simulink model "dev_AON_AOF_custom_detection_s_works"  (R2017b)
settings: Solver=ode5  StartTime=0.0  StopTime=20  FixedStep=0.025  RelTol=1e-3  EnableMultiTasking=on
undefined symbols (not defined in the file or in its folder): A1, B1
libraries: simulink x3
settings Model: Creator=b1048743  LastModifiedBy=Tom
settings DataIOCC: LimitDataPoints=on  SaveFormat=Array  SignalLoggingSaveFormat=ModelDataLogs  SignalLoggingName=sigsOut
settings OptimizationCC: BlockReduction=off  BooleanDataType=off
settings DebuggingCC: SaveWithParameterizedLinksMsg=none  UnderspecifiedInitializationDetection=Classic  MergeDetectMultiDrivingBlocksExec=none  SignalResolutionControl=TryResolveAllWithWarning  MultiTaskDSMMsg=warning  MultiTaskCondExecSysMsg=none
settings HardwareCC: ProdBitPerPointer=32  ProdBitPerSizeT=32  ProdBitPerPtrDiffT=32  ProdLargestAtomicFloat=None  ProdIntDivRoundTo=Undefined  ProdEndianess=Unspecified  ProdWordSize=32  ProdHWDeviceType=32-bit Generic  TargetUnknown=on
settings ModelReferenceCC: PropagateSignalLabelsOutOfModel=off
settings CodeAppCC: StateflowObjectComments=on
settings GRTTargetCC: TargetLangStandard=C89/C90 (ANSI)  CombineOutputUpdateFcns=off  GRTInterface=on
settings ConfigComp: CovMetricSettings=dw  CovHtmlReporting=on  CovSaveCumulativeToWorkspaceVar=on  CovSaveSingleToWorkspaceVar=on  CovExternalEMLEnable=off

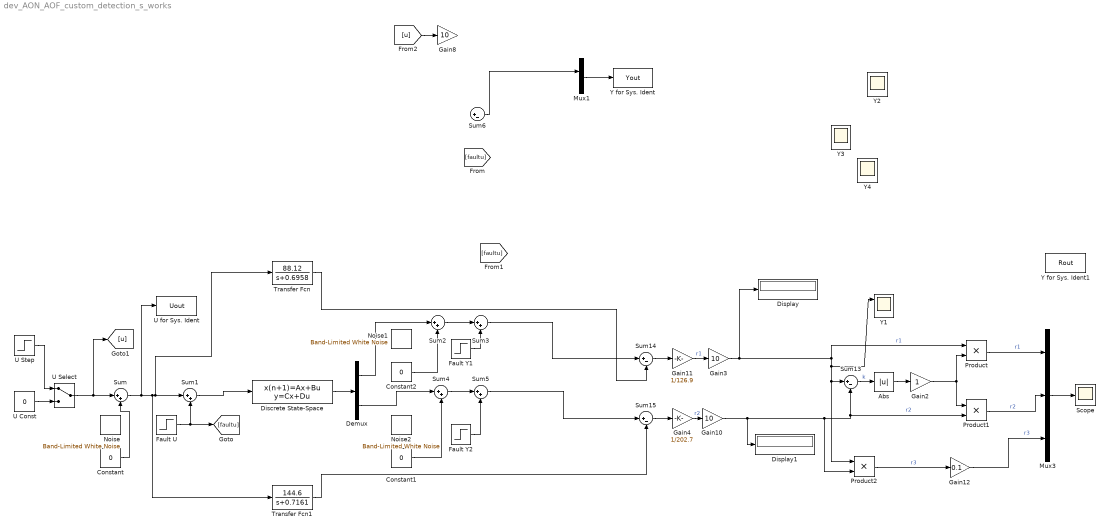
== system dev_AON_AOF_custom_detection_s_works ==
  Abs : Abs
  Constant : Constant  Value=0
  Constant1 : Constant  Value=0
  Constant2 : Constant  Value=0
  Demux : Demux  Outputs=2
  Discrete State-Space : DiscreteStateSpace  A=A1  B=B1  C=[1 0; 0 1]  D=[0;0]  SampleTime=0.025
  Display : Display
  Display1 : Display
  Fault U : Step  Time=10  After=10  SampleTime=0
  Fault Y1 : Step  Time=10  After=0  SampleTime=0
  Fault Y2 : Step  Time=10  After=0  SampleTime=0
  Gain10 : Gain  Gain=10
  Gain11 : Gain  Gain=1/126.9
  Gain12 : Gain  Gain=0.1
  Gain2 : Gain
  Gain3 : Gain  Gain=10
  Gain4 : Gain  Gain=1/202.7
  Gain8 : Gain  Gain=10
  Mux1 : Mux
  Mux3 : Mux  Inputs=3
  Noise : simulink/Sources/Band-Limited White Noise  Cov=[0.01]  Ts=0.025  seed=[23341]
  Noise1 : simulink/Sources/Band-Limited White Noise  Cov=[0.1]  Ts=0.025  seed=[23341]
  Noise2 : simulink/Sources/Band-Limited White Noise  Cov=[0.1]  Ts=0.025  seed=[23341]
  Product : Product
  Product1 : Product
  Product2 : Product
  Scope : Scope
  Sum{,1..5} (6 alike) : Sum  Inputs=|++  SaturateOnIntegerOverflow=on
  Sum{6,13..15} (4 alike) : Sum  Inputs=|+-
  Transfer Fcn : TransferFcn  Numerator=[88.12]  Denominator=[1 0.6958]
  Transfer Fcn1 : TransferFcn  Numerator=[144.6]  Denominator=[1 0.7161]
  U Const : Constant  Value=0
  "U Select " : ManualSwitch
  U Step : Step  SampleTime=0
  U for Sys. Ident : ToWorkspace  VariableName=Uout  SampleTime=0.025
  Y for Sys. Ident : ToWorkspace  VariableName=Yout  SampleTime=0.025
  Y for Sys. Ident1 : ToWorkspace  VariableName=Rout  SampleTime=0.025
  Y1 : Scope  NumInputPorts=3
  Y2 : Scope  NumInputPorts=3
  Y3 : Scope
  Y4 : Scope
  wires:
  U Const/1 -> "U Select "/2
  U Step/1 -> "U Select "/1
  Mux1/1 -> Y for Sys. Ident/1
  Discrete State-Space/1 -> Demux/1
  Sum1/1 -> Discrete State-Space/1
  Fault U/1 -> [faultu], Sum1/2
  Sum2/1 -> Sum3/1
  Fault Y1/1 -> Sum3/2
  Sum4/1 -> Sum5/1
  Fault Y2/1 -> Sum5/2
  Demux/1 -> Sum2/1
  Demux/2 -> Sum4/1
  "U Select "/1 -> [u], Sum/1
  Sum6/1 -> Mux1/2
  Constant/1 -> Sum/2
  Constant1/1 -> Sum4/2
  [u] -> Gain8/1
  Transfer Fcn1/1 -> Sum15/2
  Product/1 -> Mux3/1  "r1"
  Sum14/1 -> Gain11/1
  Sum13/1 -> Abs/1  "k"
  Gain10/1 -> Display1/1, Sum13/2, Product1/2, Product2/2  "r2"
  Gain2/1 -> Product/2, Product1/1
  Gain3/1 -> Display/1, Product/1, Y1/1, Product2/1, Sum13/1  "r1"
  Mux3/1 -> Scope/1
  Sum5/1 -> Sum15/1
  Gain12/1 -> Mux3/3  "r3"
  Transfer Fcn/1 -> Sum14/2
  Sum3/1 -> Sum14/1
  Product1/1 -> Mux3/2  "r2"
  Sum15/1 -> Gain4/1
  Sum/1 -> Transfer Fcn/1, Sum1/1, Transfer Fcn1/1, U for Sys. Ident/1
  Constant2/1 -> Sum2/2
  Product2/1 -> Gain12/1  "r3"
  Abs/1 -> Gain2/1
  Gain4/1 -> Gain10/1  "r2"
  Gain11/1 -> Gain3/1  "r1"
